simulink model "IO_sim"  (R2023b)
settings: Solver=VariableStepAuto  StartTime=0.0  StopTime=10  RelTol=1e-3
values from neighbouring files (symbols this model uses):
  x0 = [3 5]'    [IO_linearization.m]
settings Model: Creator=claudio  LastModifiedBy=stefa
settings OptimizationCC: ReuseModelBlockBuffer=off

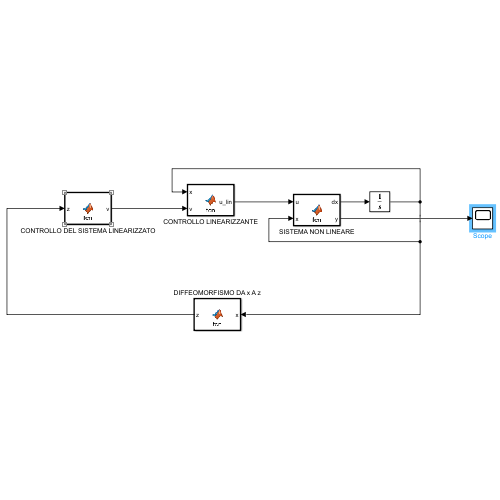
[thumbnail: Simulink's stored preview of the top-level diagram]
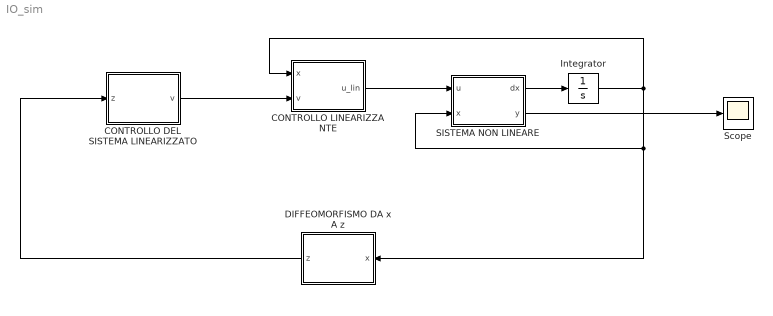
== system IO_sim ==
  CONTROLLO DEL SISTEMA LINEARIZZATO : MATLAB Function  TreatAsAtomicUnit=on
  CONTROLLO LINEARIZZANTE : MATLAB Function  TreatAsAtomicUnit=on
  DIFFEOMORFISMO DA x A z : MATLAB Function  TreatAsAtomicUnit=on
  Integrator : Integrator  InitialCondition=x0
  SISTEMA NON LINEARE : MATLAB Function  TreatAsAtomicUnit=on
  Scope : Scope
  wires:
  SISTEMA NON LINEARE/1(dx) -> Integrator/1
  Integrator/1 -> DIFFEOMORFISMO DA x A z/1(x), SISTEMA NON LINEARE/2(x), CONTROLLO LINEARIZZANTE/1(x)
  CONTROLLO LINEARIZZANTE/1(u_lin) -> SISTEMA NON LINEARE/1(u)
  CONTROLLO DEL SISTEMA LINEARIZZATO/1(v) -> CONTROLLO LINEARIZZANTE/2(v)
  DIFFEOMORFISMO DA x A z/1(z) -> CONTROLLO DEL SISTEMA LINEARIZZATO/1(z)
  SISTEMA NON LINEARE/2(y) -> Scope/1

== matlab function IO_sim/SISTEMA NON LINEARE ==
  data: u input; dx output; x input; y output
function [dx,y]= fcn(u,x)

x1=x(1);
x2=x(2);
dx=[(x1^2+x1)*x2;-2*x2+x1-x2*u+6*u];
y=5*x1;

== matlab function IO_sim/CONTROLLO DEL SISTEMA LINEARIZZATO ==
  data: z input; v output
function v = fcn(z)
z1=z(1);
z2=z(2);
K=[ 50 15] % risultato del comando place
v=-K(1)*z1-K(2)*z2; % avrei potuto scrivere -K*z

== matlab function IO_sim/DIFFEOMORFISMO DA x A z ==
  data: x input; z output
function z = fcn(x)
x1=x(1);
x2=x(2);
z=[5*x1;5*x2*(x1^2 + x1)];

== matlab function IO_sim/CONTROLLO LINEARIZZANTE ==
  data: x input; v input; u_lin output
function u_lin = fcn(x,v)
x1=x(1);
x2=x(2);
u_lin=((5*x1^2 + 5*x1)*(x1 - 2*x2) - v + 5*x2^2*(2*x1 + 1)*(x1^2 + x1))/((5*x1^2 + 5*x1)*(x2 - 6));
